simulink model "send_pressure_udp"  (R2018a)
settings: Solver=ode4  StartTime=0.0  StopTime=inf  FixedStep=0.005  RelTol=1e-3  EnableMultiTasking=on
PostLoadFcn:
  | qc_set_target_type(getConfigSet(bdroot, 'QUARC Default Target Configuration'));
InitFcn:
  | dataSave_0 = 0
  | dataSave_1 = 0
  | dataSave_2 = 0
undefined symbols (not defined in the file or in its folder): HIL
libraries: quarc_library x4, dspstat3 x3, dspnetwork x1
Description:
  | This example is a simple analog loopback test. It sends a signal to analog output
  | channel #0 and then reads analog input channel #0. Wire analog output #0 to analog
  | input #0 to see the signal on the Scope. Change the amplitude of the signal and see
  | the change occur on the Scope.
settings Model: SimulationMode=external  ExtModeTrigDuration=10000  Creator=drmadill  LastModifiedBy=dogro
settings SolverCC: PositivePriorityOrder=on
settings DataIOCC: LimitDataPoints=on  SaveFormat=Array  SignalLoggingSaveFormat=ModelDataLogs
settings OptimizationCC: ExpressionDepthLimit=2147483647  InitFltsAndDblsToZero=on  LifeSpan=inf
settings DebuggingCC: SaveWithParameterizedLinksMsg=none  SolverPrmCheckMsg=warning  FcnCallInpInsideContextMsg=warning  StateNameClashWarn=warning  SFUnexpectedBacktrackingDiag=warning  SFNoUnconditionalDefaultTransitionDiag=warning  SFExecutionAtInitializationDiag=none
settings HardwareCC: ProdBitPerPointer=32  ProdBitPerSizeT=32  ProdBitPerPtrDiffT=32  ProdLargestAtomicFloat=None  ProdIntDivRoundTo=Undefined  ProdEndianess=Unspecified  ProdWordSize=32  ProdHWDeviceType=32-bit Generic
settings ModelReferenceCC: PropagateSignalLabelsOutOfModel=off
settings RTWCC: SystemTargetFile=quarc_win64.tlc  TemplateMakefile=quarc_default_tmf  Description=QUARC Win64 Target
settings CodeAppCC: StateflowObjectComments=on
settings STFCustomTargetCC: TargetPreCompLibLocation=C:\PROGRA~3\QUARC\lib\2018a\win64\release  ConcurrentExecutionCompliant=on  GeneratePreprocessorConditionals=Disable all  CPPClassGenCompliant=on  SystemTargetFile=quarc_win64.tlc
settings GRTTargetCC: TargetPreCompLibLocation=C:\PROGRA~3\QUARC\lib\2018a\win64\release  TargetLangStandard=C89/C90 (ANSI)  ParMdlRefBuildCompliant=off  CompOptLevelCompliant=off  GeneratePreprocessorConditionals=Disable all  CombineOutputUpdateFcns=off  MatFileLogging=off  GRTInterface=on  UseToolchainInfoCompliant=off  ExtMode=on  ExtModeMexFile=quarc_comm
settings ConfigComp: CovMetricSettings=dw  CovHtmlReporting=on  CovSaveCumulativeToWorkspaceVar=on  CovSaveSingleToWorkspaceVar=on  CovExternalEMLEnable=off

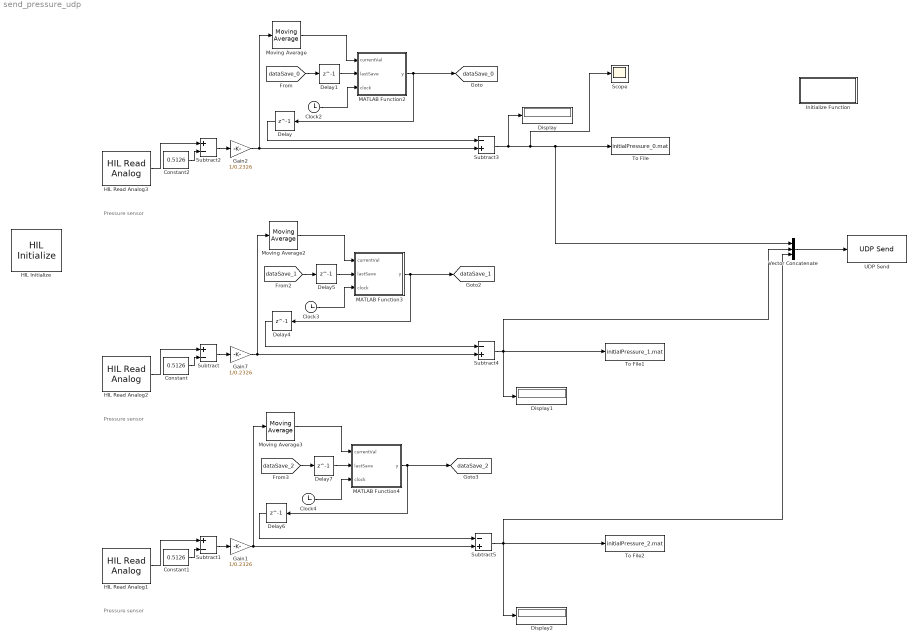
== system send_pressure_udp ==
  note: Pressure sensor
  note: Pressure sensor
  note: Pressure sensor
  Clock2 : Clock
  Clock3 : Clock
  Clock4 : Clock
  Constant : Constant  Value=0.5126
  Constant1 : Constant  Value=0.5126
  Constant2 : Constant  Value=0.5126
  Delay{,1,4..7} (6 alike) : Delay  DelayLength=1
  Display : Display
  Display1 : Display
  Display2 : Display
  Gain1 : Gain  Gain=1/0.2326
  Gain2 : Gain  Gain=1/0.2326
  Gain7 : Gain  Gain=1/0.2326
  HIL Initialize : quarc_library/Data Acquisition/Generic/Configuration/HIL Initialize  Priority=-99  object_name=HIL-1  board_type=qpid_e  board_number=0  board_options=enc0_dir=0;enc0_filter=1;enc0_a=1;enc0_b=1;enc0_z=0;enc0_reload=0;enc1_dir=0;enc1_filter=1;enc1_a=1;enc1_b=1;enc1_z=0;enc1_reload=0;enc2_dir=0;enc2_filter=1;enc2_a=1;enc2_b=1;enc2_z=0;enc2_reload=0;enc3_dir=0;enc3_filter=1;enc3_a=1;enc3_b=1;enc3_z=0;enc3_reload=0;enc4_dir=0;enc4_filter=1;enc4_a=1;enc4_b=1;enc4_z=0;enc4_reload=0;enc5_dir=0;enc5_filter=1;enc5_a=1;enc5_b=1;enc5_z=0;enc5_reload=0;enc6_dir=0;enc6_filter=1;enc6_a=1;enc6_b=1;enc6_z=0;enc6_reload=0;enc7_dir=0;enc7_filter=1;enc7_a=1;enc7_b=1;enc7_z=0;enc7_reload=0;ext_int_polarity=0;fuse_polarity=0;convert_polarity=0;watchdog_polarity=0;ext_int_watchdog=0;fuse_watchdog=0;trig1_watchdog=0;watchdog_to_trig1=0;watchdog_to_trig2=0;counter_to_trig0=0;trigger_adcs=0;latch_on_adc=0;pwm_immediate=0  exclusive=off  active=off  hardware_clocks=[0:16]  clock_modes=[]  initial_clock_frequencies=[]  set_clock_params_at_start=off  set_clock_params_at_switch_in=off  set_clock_frequencies_at_start=off  set_clock_frequencies_at_switch_in=off  analog_input_channels=[0:7]  analog_input_configurations=[]  analog_input_maximums=10  analog_input_minimums=-10  set_analog_input_params_at_start=off  set_analog_input_params_at_switch_in=off  analog_output_channels=[0:7]  analog_output_maximums=10  analog_output_minimums=-10  initial_analog_outputs=[0]  final_analog_outputs=[0]  watchdog_analog_outputs=0  set_analog_output_params_at_start=off  set_analog_output_params_at_switch_in=off  set_analog_outputs_at_start=on  set_analog_outputs_at_switch_in=off  set_analog_outputs_at_terminate=on  set_analog_outputs_at_switch_out=off  set_analog_outputs_on_watchdog=off  digital_input_channels=[]  digital_output_channels=[]  digital_output_configuration=[]  initial_digital_outputs=[1]  final_digital_outputs=[1]  watchdog_digital_outputs=[2]  set_digital_output_params_at_start=off  set_digital_output_params_at_switch_in=off  set_digital_outputs_at_start=on  set_digital_outputs_at_switch_in=off  set_digital_outputs_at_terminate=on  set_digital_outputs_at_switch_out=off  set_digital_outputs_on_watchdog=off  encoder_channels=[0:7]  quadrature=[4]  encoder_filter_frequency=40e6/1  initial_encoder_counts=[0]  set_encoder_params_at_start=on  set_encoder_params_at_switch_in=off  set_encoder_counts_at_start=on  set_encoder_counts_at_switch_in=off  pwm_channels=[0:7]  pwm_modes=0  pwm_frequency=40e6/4096  pwm_configuration=[0]  pwm_alignment=[0]  pwm_polarity=[1]  pwm_leading_deadband=[0]  pwm_trailing_deadband=[0]  initial_pwm_outputs=[0]  final_pwm_outputs=[0]  watchdog_pwm_outputs=[0]  set_pwm_params_at_start=on  set_pwm_params_at_switch_in=off  set_pwm_outputs_at_start=on  set_pwm_outputs_at_switch_in=off  set_pwm_outputs_at_terminate=on  set_pwm_outputs_at_switch_out=off  set_pwm_outputs_on_watchdog=off  other_output_channels=[]  initial_other_outputs=[]  final_other_outputs=[]  watchdog_other_outputs=[]  set_other_outputs_at_start=off  set_other_outputs_at_switch_in=off  set_other_outputs_at_terminate=off  set_other_outputs_at_switch_out=off  set_other_outputs_on_watchdog=off
  HIL Read Analog1 : quarc_library/Data Acquisition/Generic/Immediate I//O/HIL Read Analog  object_name=HIL-1  channels=[2]  sample_time=qc_get_step_size  active=on  vector_output=off
  HIL Read Analog2 : quarc_library/Data Acquisition/Generic/Immediate I//O/HIL Read Analog  object_name=HIL-1  channels=[3]  sample_time=qc_get_step_size  active=on  vector_output=off
  HIL Read Analog3 : quarc_library/Data Acquisition/Generic/Immediate I//O/HIL Read Analog  object_name=HIL-1  channels=[0]  sample_time=qc_get_step_size  active=on  vector_output=off
  Initialize Function : Subsystem  TreatAsAtomicUnit=on
  MATLAB Function2 : MATLAB Function  TreatAsAtomicUnit=on
  MATLAB Function3 : MATLAB Function  TreatAsAtomicUnit=on
  MATLAB Function4 : MATLAB Function  TreatAsAtomicUnit=on
  Moving Average : dspstat3/Moving Average  Method=Sliding window  ForgettingFactorPort=off  SpecifyWindowLength=on  WindowLength=200  ForgettingFactor=0.9  SimulateUsing=Code generation
  Moving Average2 : dspstat3/Moving Average  Method=Sliding window  ForgettingFactorPort=off  SpecifyWindowLength=on  WindowLength=200  ForgettingFactor=0.9  SimulateUsing=Code generation
  Moving Average3 : dspstat3/Moving Average  Method=Sliding window  ForgettingFactorPort=off  SpecifyWindowLength=on  WindowLength=200  ForgettingFactor=0.9  SimulateUsing=Code generation
  Scope : Scope
  Subtract : Sum  Inputs=+-
  Subtract1 : Sum  Inputs=+-
  Subtract2 : Sum  Inputs=+-
  Subtract3 : Sum  Inputs=-+
  Subtract4 : Sum  Inputs=-+
  Subtract5 : Sum  Inputs=-+
  To File : ToFile  Filename=initialPressure_0.mat
  To File1 : ToFile  Filename=initialPressure_1.mat
  To File2 : ToFile  Filename=initialPressure_2.mat
  UDP Send : dspnetwork/UDP Send  remoteURL='127.0.0.1'  remotePort=25000  localURL='0.0.0.0'  localPortSource=Automatically determine  localPort=-1  sampletime=-1  blockPlatform=[]  separateLengthPort=0
      settings: SourceProductName=DSP System Toolbox  SourceProductBaseCode=DS
  Vector Concatenate : Concatenate  NumInputs=3  Mode=Multidimensional array
  tag scope: dataSave_0=global, dataSave_1=global, dataSave_2=global
  wires:
  HIL Read Analog2/1 -> Subtract/1
  Subtract/1 -> Gain7/1
  Constant/1 -> Subtract/2
  Subtract1/1 -> Gain1/1
  HIL Read Analog1/1 -> Subtract1/1
  Constant1/1 -> Subtract1/2
  Subtract2/1 -> Gain2/1
  HIL Read Analog3/1 -> Subtract2/1
  Constant2/1 -> Subtract2/2
  Vector Concatenate/1 -> UDP Send/1
  Subtract3/1 -> Scope/1, Vector Concatenate/1, To File/1, Display/1
  Gain2/1 -> Subtract3/2, Moving Average/1
  Gain7/1 -> Subtract4/2, Moving Average2/1
  Subtract4/1 -> Display1/1, To File1/1, Vector Concatenate/2
  Subtract5/1 -> Display2/1, To File2/1, Vector Concatenate/3
  Clock2/1 -> MATLAB Function2/3(clock)
  MATLAB Function2/1(y) -> Delay/1, [dataSave_0]
  Moving Average/1 -> MATLAB Function2/1(currentVal)
  [dataSave_0] -> Delay1/1
  Delay1/1 -> MATLAB Function2/2(lastSave)
  Clock3/1 -> MATLAB Function3/3(clock)
  MATLAB Function3/1(y) -> Delay4/1, [dataSave_1]
  [dataSave_1] -> Delay5/1
  Delay5/1 -> MATLAB Function3/2(lastSave)
  Moving Average2/1 -> MATLAB Function3/1(currentVal)
  Clock4/1 -> MATLAB Function4/3(clock)
  MATLAB Function4/1(y) -> Delay6/1, [dataSave_2]
  [dataSave_2] -> Delay7/1
  Moving Average3/1 -> MATLAB Function4/1(currentVal)
  Delay7/1 -> MATLAB Function4/2(lastSave)
  Delay/1 -> Subtract3/1
  Delay4/1 -> Subtract4/1
  Gain1/1 -> Moving Average3/1, Subtract5/2
  Delay6/1 -> Subtract5/1

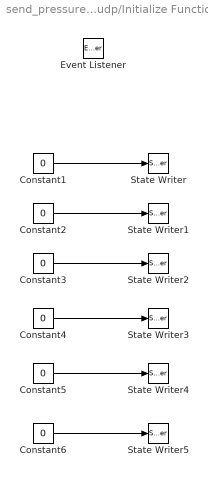
== system send_pressure_udp/Initialize Function ==
  Constant{1..6} (6 alike) : Constant  Value=0
  Event Listener : EventListener  DisableCoverage=on  EventName=reset
  State Writer : StateWriter  StateOwnerBlock=../../Delay
  State Writer1 : StateWriter  StateOwnerBlock=../../Delay1
  State Writer2 : StateWriter  StateOwnerBlock=../../Delay4
  State Writer3 : StateWriter  StateOwnerBlock=../../Delay5
  State Writer4 : StateWriter  StateOwnerBlock=../../Delay6
  State Writer5 : StateWriter  StateOwnerBlock=../../Delay7
  wires:
  Constant1/1 -> State Writer/1
  Constant2/1 -> State Writer1/1
  Constant3/1 -> State Writer2/1
  Constant4/1 -> State Writer3/1
  Constant5/1 -> State Writer4/1
  Constant6/1 -> State Writer5/1

== matlab function send_pressure_udp/MATLAB Function2 ==
  data: currentVal input; lastSave input; y output; clock input
function y = fcn(currentVal,lastSave,clock)

if clock < 10
    y = currentVal;
else y = lastSave;
    
clock
currentVal
lastSave

end

== matlab function send_pressure_udp/MATLAB Function3 ==
  data: currentVal input; lastSave input; y output; clock input
function y = fcn(currentVal,lastSave,clock)

if clock < 10
    y = currentVal;
else y = lastSave;
    
clock
currentVal
lastSave

end

== matlab function send_pressure_udp/MATLAB Function4 ==
  data: currentVal input; lastSave input; y output; clock input
function y = fcn(currentVal,lastSave,clock)

if clock < 10
    y = currentVal;
else y = lastSave;
    
clock
currentVal
lastSave

end
